simulink model "hardwareModel_6FBLCtry"  (R2023b)
settings: Solver=FixedStepAuto  StartTime=0.0  StopTime=inf  RelTol=1e-3  EnableMultiTasking=on
model workspace (MAT data in the model file):
  Ts = Simulink.Parameter
  Ts.Value = 0.01
  Ts.DataType = 'auto'
  Ts.Complexity = 'real'
  Ts.Dimensions = [1 1]
values from neighbouring files (symbols this model uses):
  g = 9.80665    [modelparam.m]
  I_r_A = I_r_B + m_r*l_AB^2    (= 0.00169018666667)    [modelparam.m]
  I_w_A = I_w_C + m_w*l_AC^2    (= 0.001261425)    [modelparam.m]
  I_w_C = 0.5*m_w*R^2    (= 8.6875e-05)    [modelparam.m]
  l_AB = l/2    (= 0.065)    [modelparam.m]
  l_AC = l    (= 0.13)    [modelparam.m]
  m_r = 0.2948    [modelparam.m]
  m_w = 0.0695    [modelparam.m]
libraries: arduinomotorcarrierlib x4, simulink x1, eeGeneralControl x1, arduinosensorlib x1
settings Model: SimulationMode=external  ExtModeTrigDuration=2  Creator=bkhusain  LastModifiedBy=anura
settings SolverCC: AlgebraicLoopSolver=TrustRegion
settings OptimizationCC: EnhancedBackFolding=on  PassReuseOutputArgsThreshold=0  MaxStackSize=64  OptimizeBlockOrder=speed  DifferentSizesBufferReuse=on  OptimizationCustomize=off
settings DebuggingCC: ParameterTunabilityLossMsg=error  UnconnectedInputMsg=warning  UnconnectedOutputMsg=warning  UnconnectedLineMsg=warning
settings HardwareCC: ProdBitPerPointer=32  ProdBitPerSizeT=32  ProdBitPerPtrDiffT=32  ProdLargestAtomicInteger=Long  ProdLargestAtomicFloat=Double  ProdWordSize=32  ProdHWDeviceType=ARM Compatible->ARM Cortex  UseEmbeddedCoderFeatures=off  UseSimulinkCoderFeatures=off
settings ModelReferenceCC: EnableRefExpFcnMdlSchedulingChecks=on
settings SFSimCC: MATLABDynamicMemAlloc=off
settings RTWCC: Description=Embedded Coder  SystemTargetFile=ert.tlc  HardwareBoard=Arduino Nano 33 IoT  TemplateMakefile=ert_default_tmf  RTWVerbose=off  Toolchain=Arduino ARM  BuildConfiguration=Faster Runs
settings CodeAppCC: ForceParamTrailComments=on  OperatorAnnotations=on  MangleLength=10
settings ERTTargetCC: ERTCustomFileBanners=off  SupportContinuousTime=on  SupportNonInlinedSFcns=on  RemoveResetFunc=off  SupportVariableSizeSignals=on  ModelStepFunctionPrototypeControlCompliant=off  ExtMode=on  ExtModeTransport=3  ExtModeStaticAlloc=on  ExtModeStaticAllocSize=8192  ExtModeMexFile=ext_xcp  ExtModeMexArgs=0 7 921600  ExtModeIntrfLevel=Level2 - Open  ERTSrcFileBannerTemplate=codertarget_code_template.cgt  ERTHdrFileBannerTemplate=codertarget_code_template.cgt  ERTDataSrcFileTemplate=codertarget_code_template.cgt  ERTDataHdrFileTemplate=codertarget_code_template.cgt

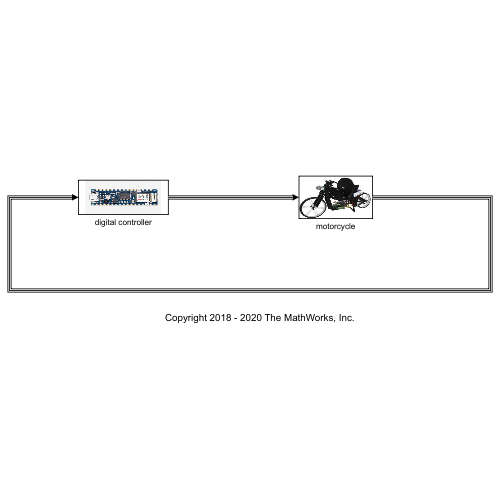
[thumbnail: Simulink's stored preview of the top-level diagram]
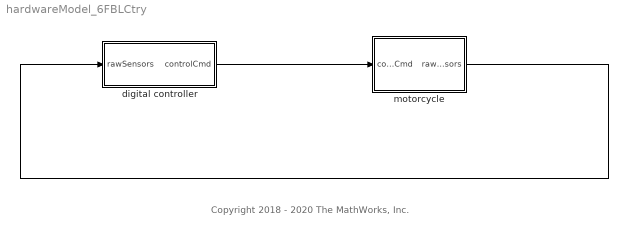
== system hardwareModel_6FBLCtry ==
  note: Copyright 2018 - 2020 The MathWorks, Inc.
  digital controller : Subsystem
      mask Display: image('$imagefile'); % Use "Edit Image" on toolstrip to change.
  motorcycle : Subsystem
      mask Display: image('$imagefile'); % Use "Edit Image" on toolstrip to change.
  wires:
  motorcycle/1(rawSensors) -> digital controller/1(rawSensors)
  digital controller/1(controlCmd) -> motorcycle/1(controlCmd)

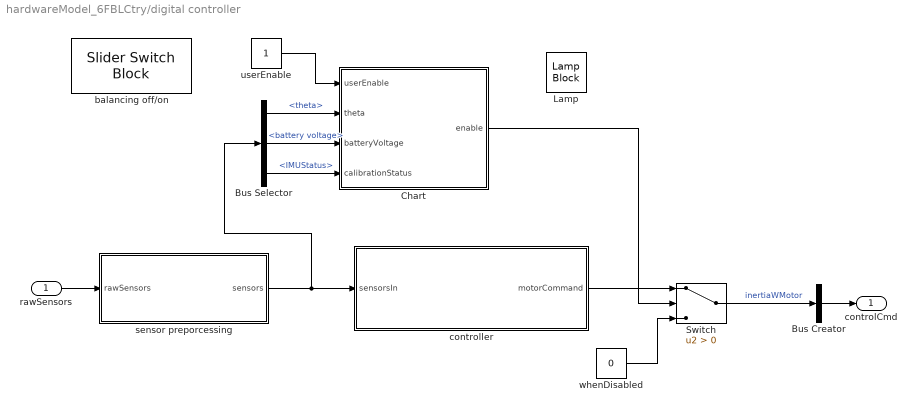
== system hardwareModel_6FBLCtry/digital controller ==
  rawSensors : Inport
  Bus Creator : BusCreator  Inputs=1
  Bus Selector : BusSelector  OutputSignals=theta,battery voltage,IMUStatus
  Chart : Stateflow chart  TreatAsAtomicUnit=on
  Lamp : LampBlock
  Switch : Switch  Criteria=u2 > Threshold  SaturateOnIntegerOverflow=off  InputSameDT=off
  balancing off/on : SliderSwitchBlock  LabelPosition=Hide
      settings: Values={{'Off', 'On'}, [0 1]}
  controller : Subsystem
  sensor preporcessing : Subsystem
  userEnable : Constant  SampleTime=Ts
  whenDisabled : Constant  Value=0  SampleTime=Ts
  controlCmd : Outport
  wires:
  Switch/1 -> Bus Creator/1  "inertiaWMotor"
  Bus Creator/1 -> controlCmd/1
  rawSensors/1 -> sensor preporcessing/1(rawSensors)
  sensor preporcessing/1(sensors) -> Bus Selector/1, controller/1(sensorsIn)
  whenDisabled/1 -> Switch/3
  Chart/1(enable) -> Switch/2
  Bus Selector/1 -> Chart/2(theta)  "<theta>"
  Bus Selector/2 -> Chart/3(batteryVoltage)  "<battery voltage>"
  Bus Selector/3 -> Chart/4(calibrationStatus)  "<IMUStatus>"
  userEnable/1 -> Chart/1(userEnable)
  controller/1(motorCommand) -> Switch/1

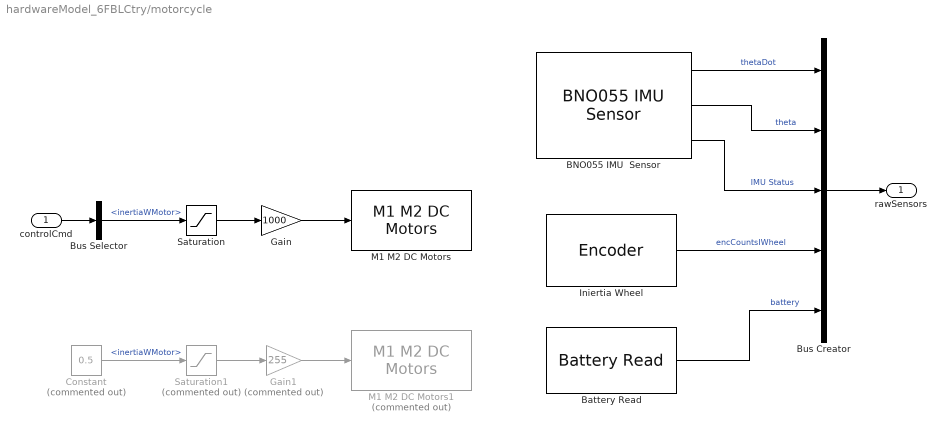
== system hardwareModel_6FBLCtry/motorcycle ==
  controlCmd : Inport
  BNO055 IMU  Sensor : arduinosensorlib/BNO055 IMU Sensor  SlaveAddress=0x28  OperationMode=Fusion  Accel=off  AngularRate=on  MagField=off  EulerAngles=on  Quat=off  LinearAccel=off  GravityVector=off  Status=on  Timestamp=off  AccelRange=4G  AccelBW=62.5 Hz  GyroRange=2000 dps  GyroBW=32 Hz  MagODR=10 Hz  spf=1  SampleTime=Ts  blockPlatform=ARDUINO  QueueSizeFactor=1
  Battery Read : arduinomotorcarrierlib/Battery Read  SlaveAddress=uint8( hex2dec( '66' ) )  blockPlatform=ARDUINO  SampleTime=Ts
  Bus Creator : BusCreator  Inputs=5
  Bus Selector : BusSelector  OutputSignals=inertiaWMotor
  Constant : Constant  Commented=on  Value=0.5
  Gain : Gain  Gain=1000
  Gain1 : Gain  Commented=on  Gain=255
  Iniertia Wheel : arduinomotorcarrierlib/Encoder  SlaveAddress=uint8( hex2dec( '66' ) )  blockPlatform=ARDUINO  Encoder=1  ShowSpeed=off  ResetOption=on  SampleTime=Ts
  M1 M2 DC Motors : arduinomotorcarrierlib/M1 M2 DC Motors  SlaveAddress=uint8( hex2dec( '66' ) )  blockPlatform=ARDUINO  MotorNumber=M1  MotorCarrierPWMFreq=100
  M1 M2 DC Motors1 : arduinomotorcarrierlib/M1 M2 DC Motors  Commented=on  SlaveAddress=uint8( hex2dec( '66' ) )  blockPlatform=ARDUINO  MotorNumber=M2  MotorCarrierPWMFreq=100
  Saturation : Saturate  UpperLimit=100  LowerLimit=-100
  Saturation1 : Saturate  Commented=on  UpperLimit=100  LowerLimit=-100
  rawSensors : Outport
  wires:
  BNO055 IMU  Sensor/1 -> Bus Creator/1  "thetaDot"
  BNO055 IMU  Sensor/2 -> Bus Creator/2  "theta"
  BNO055 IMU  Sensor/3 -> Bus Creator/3  "IMU Status"
  Iniertia Wheel/1 -> Bus Creator/4  "encCountsIWheel"
  Battery Read/1 -> Bus Creator/5  "battery"
  Bus Creator/1 -> rawSensors/1
  controlCmd/1 -> Bus Selector/1
  Bus Selector/1 -> Saturation/1  "<inertiaWMotor>"
  Constant/1 -> Saturation1/1  "<inertiaWMotor>"
  Saturation1/1 -> Gain1/1
  Gain1/1 -> M1 M2 DC Motors1/1
  Gain/1 -> M1 M2 DC Motors/1
  Saturation/1 -> Gain/1

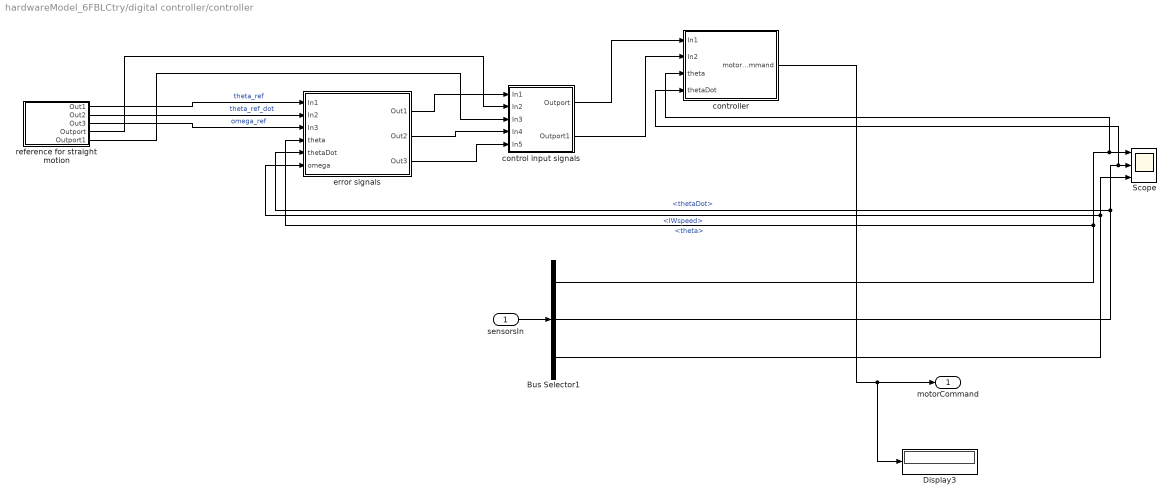
== system hardwareModel_6FBLCtry/digital controller/controller ==
  sensorsIn : Inport
  Bus Selector1 : BusSelector  OutputSignals=theta,thetaDot,IWspeed
  Display3 : Display
  Scope : Scope  NumInputPorts=3
  control input signals : Subsystem
  controller : Subsystem
  error signals : Subsystem
  reference for straight motion : Subsystem
  motorCommand : Outport
  wires:
  sensorsIn/1 -> Bus Selector1/1
  reference for straight motion/3(Out3) -> error signals/3(In3)  "omega_ref"
  reference for straight motion/2(Out2) -> error signals/2(In2)  "theta_ref_dot"
  reference for straight motion/1(Out1) -> error signals/1(In1)  "theta_ref"
  error signals/2(Out2) -> control input signals/4(In4)
  error signals/3(Out3) -> control input signals/5(In5)
  reference for straight motion/4(Outport) -> control input signals/2(In2)
  reference for straight motion/5(Outport1) -> control input signals/3(In3)
  error signals/1(Out1) -> control input signals/1(In1)
  control input signals/2(Outport1) -> controller/2(In2)
  Bus Selector1/2 -> controller/4(thetaDot), Scope/2, error signals/5(thetaDot)  "<thetaDot>"
  Bus Selector1/3 -> Scope/3, error signals/6(omega)  "<IWspeed>"
  Bus Selector1/1 -> controller/3(theta), Scope/1, error signals/4(theta)  "<theta>"
  control input signals/1(Outport) -> controller/1(In1)
  controller/1(motorCommand) -> Display3/1, motorCommand/1

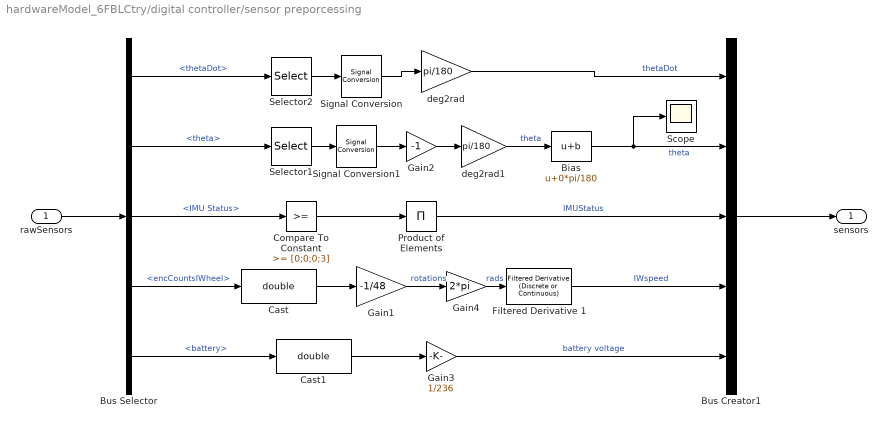
== system hardwareModel_6FBLCtry/digital controller/sensor preporcessing ==
  rawSensors : Inport
  Bias : Bias  Bias=0*pi/180  SaturateOnIntegerOverflow=off
  Bus Creator1 : BusCreator  Inputs=5
  Bus Selector : BusSelector  OutputSignals=thetaDot,theta,IMU Status,encCountsIWheel,battery
  Cast : DataTypeConversion  OutDataTypeStr=double  SaturateOnIntegerOverflow=off  RndMeth=Floor
  Cast1 : DataTypeConversion  OutDataTypeStr=double  SaturateOnIntegerOverflow=off  RndMeth=Floor
  Compare To Constant : simulink/Logic and Bit Operations/Compare To Constant  relop=>=  const=[0;0;0;3]  OutDataTypeStr=boolean
  Filtered Derivative 1 : eeGeneralControl/Filtered Derivative (Discrete or Continuous)  K=1  T=0.1  B=inf  A=-inf  minRatio=10  init_option=Inherited from block input  x0=0  Ts=Ts
  Gain1 : Gain  Gain=-1/48
  Gain2 : Gain  Gain=-1
  Gain3 : Gain  Gain=1/236
  Gain4 : Gain  Gain=2*pi
  Product of Elements : Product  Inputs=*
  Scope : Scope
  Selector1 : Selector  InputPortWidth=3  IndexOptions=Index vector (dialog)  Indices=[2]  OutputSizes=1
  Selector2 : Selector  InputPortWidth=3  IndexOptions=Index vector (dialog)  Indices=[2]  OutputSizes=1
  Signal Conversion : SignalConversion  OverrideOpt=off
  Signal Conversion1 : SignalConversion  OverrideOpt=off
  deg2rad : Gain  Gain=pi/180
  deg2rad1 : Gain  Gain=pi/180
  sensors : Outport
  wires:
  Bus Selector/4 -> Cast/1  "<encCountsIWheel>"
  Compare To Constant/1 -> Product of Elements/1
  Bus Selector/5 -> Cast1/1  "<battery>"
  Selector2/1 -> Signal Conversion/1
  Bus Selector/2 -> Selector1/1  "<theta>"
  Selector1/1 -> Signal Conversion1/1
  Cast1/1 -> Gain3/1
  Bus Selector/3 -> Compare To Constant/1  "<IMU Status>"
  rawSensors/1 -> Bus Selector/1
  Product of Elements/1 -> Bus Creator1/3  "IMUStatus"
  Filtered Derivative 1/1 -> Bus Creator1/4  "IWspeed"
  deg2rad1/1 -> Bias/1  "theta"
  Bus Selector/1 -> Selector2/1  "<thetaDot>"
  Gain3/1 -> Bus Creator1/5  "battery voltage"
  Bus Creator1/1 -> sensors/1
  Signal Conversion1/1 -> Gain2/1
  Gain2/1 -> deg2rad1/1
  Signal Conversion/1 -> deg2rad/1
  Cast/1 -> Gain1/1
  Gain1/1 -> Gain4/1  "rotations"
  Gain4/1 -> Filtered Derivative 1/1  "rads"
  deg2rad/1 -> Bus Creator1/1  "thetaDot"
  Bias/1 -> Scope/1, Bus Creator1/2  "theta"

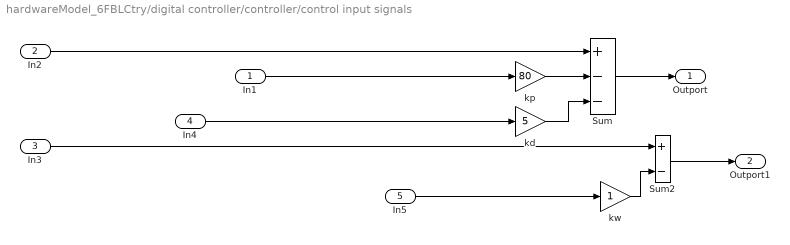
== system hardwareModel_6FBLCtry/digital controller/controller/control input signals ==
  In1 : Inport
  In2 : Inport  Port=2
  In3 : Inport  Port=3
  In4 : Inport  Port=4
  In5 : Inport  Port=5
  Sum : Sum  Inputs=+--
  Sum2 : Sum  Inputs=+-
  kd : Gain  Gain=5
  kp : Gain  Gain=80
  kw : Gain
  Outport : Outport
  Outport1 : Outport  Port=2
  wires:
  Sum/1 -> Outport/1
  In3/1 -> Sum2/1
  Sum2/1 -> Outport1/1
  In5/1 -> kw/1
  In1/1 -> kp/1
  kd/1 -> Sum/3
  kp/1 -> Sum/2
  In2/1 -> Sum/1
  kw/1 -> Sum2/2
  In4/1 -> kd/1

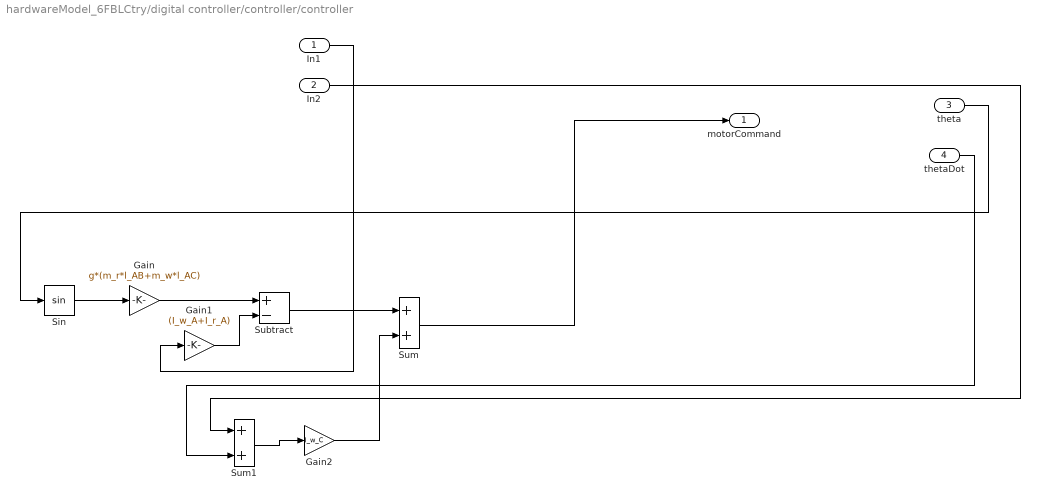
== system hardwareModel_6FBLCtry/digital controller/controller/controller ==
  In1 : Inport
  In2 : Inport  Port=2
  theta : Inport  Port=3
  thetaDot : Inport  Port=4
  Gain : Gain  Gain=g*(m_r*l_AB+m_w*l_AC)
  Gain1 : Gain  Gain=(I_w_A+I_r_A)
  Gain2 : Gain  Gain=I_w_C
  Sin : Trigonometry
  Subtract : Sum  Inputs=+-
  Sum : Sum
  Sum1 : Sum
  motorCommand : Outport
  wires:
  Subtract/1 -> Sum/1
  In1/1 -> Gain1/1
  Sum/1 -> motorCommand/1
  Gain1/1 -> Subtract/2
  Sum1/1 -> Gain2/1
  Sin/1 -> Gain/1
  thetaDot/1 -> Sum1/2
  Gain/1 -> Subtract/1
  Gain2/1 -> Sum/2
  In2/1 -> Sum1/1
  theta/1 -> Sin/1

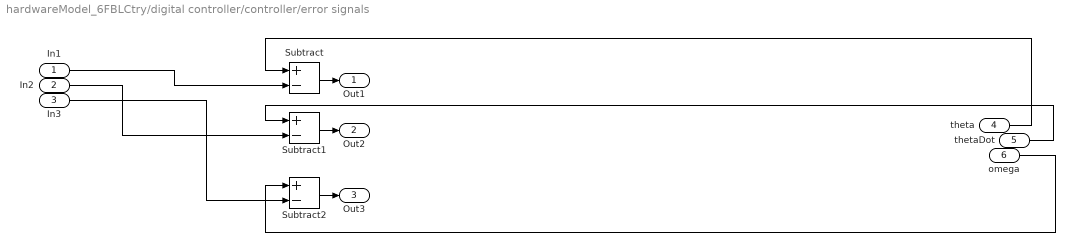
== system hardwareModel_6FBLCtry/digital controller/controller/error signals ==
  In1 : Inport
  In2 : Inport  Port=2
  In3 : Inport  Port=3
  theta : Inport  Port=4
  thetaDot : Inport  Port=5
  omega : Inport  Port=6
  Subtract : Sum  Inputs=+-
  Subtract1 : Sum  Inputs=+-
  Subtract2 : Sum  Inputs=+-
  Out1 : Outport
  Out2 : Outport  Port=2
  Out3 : Outport  Port=3
  wires:
  In1/1 -> Subtract/2
  In3/1 -> Subtract2/2
  thetaDot/1 -> Subtract1/1
  Subtract2/1 -> Out3/1
  omega/1 -> Subtract2/1
  theta/1 -> Subtract/1
  Subtract/1 -> Out1/1
  Subtract1/1 -> Out2/1
  In2/1 -> Subtract1/2

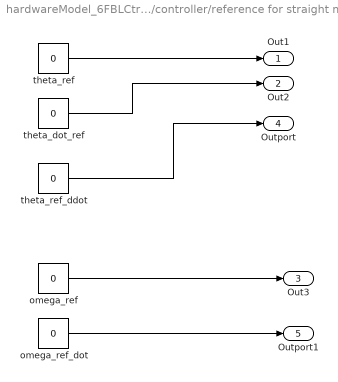
== system hardwareModel_6FBLCtry/digital controller/controller/reference for straight motion ==
  omega_ref : Constant  Value=0
  omega_ref_dot : Constant  Value=0
  theta_dot_ref : Constant  Value=0
  theta_ref : Constant  Value=0
  theta_ref_ddot : Constant  Value=0
  Out1 : Outport
  Out2 : Outport  Port=2
  Out3 : Outport  Port=3
  Outport : Outport  Port=4
  Outport1 : Outport  Port=5
  wires:
  theta_dot_ref/1 -> Out2/1
  theta_ref/1 -> Out1/1
  omega_ref/1 -> Out3/1
  theta_ref_ddot/1 -> Outport/1
  omega_ref_dot/1 -> Outport1/1

== stateflow chart hardwareModel_6FBLCtry/digital controller/Chart ==
  state checkFallen [parallel]
    settings: executionOrder=1
    state fallen
      entry: upright = false
    state standing
      entry: upright = true
    (default) -> fallen
    fallen -> standing : [abs(theta) <pi*12/180]
    standing -> fallen : [abs(theta) > pi*12/180]
  state checkIMUCalib [parallel]
    settings: executionOrder=2
    state imuNotCalibrated
      entry:
      IMUCalibrated = false;
    state imuCalibrated
      entry:
      IMUCalibrated = true;
    (default) -> imuNotCalibrated
    imuNotCalibrated -> imuCalibrated : [calibrationStatus == true]
  state checkBattery [parallel]
    settings: executionOrder=3
    state batteryNotCharged
      entry:
      batteryOK = false;
    state batteryCharged
      entry:
      batteryOK = true;
    (default) -> batteryNotCharged
    batteryCharged -> batteryNotCharged : [batteryVoltage < 3.0]
    batteryNotCharged -> batteryCharged : [batteryVoltage >= 3.0]
  state calculateEnable [parallel]
    settings: executionOrder=4
    state disableControl
      entry: enable = false
    state enableControl
      entry: enable = true
    (default) -> disableControl
    disableControl -> enableControl : [userEnable&& batteryOK && IMUCalibrated && upright]
    enableControl -> disableControl : [not(userEnable) || not(batteryOK) || not(IMUCalibrated) || not(upright)]
  data: userEnable input; theta input; enable output; batteryVoltage input; calibrationStatus input; upright local; IMUCalibrated local; batteryOK local
